simulink model "test_emplanner_cs_old"  (R2021a)
settings: Solver=ode5  StartTime=0.0  StopTime=120  FixedStep=1/1000  RelTol=1e-3
PreLoadFcn:
  | mbxruntime.callbacks.PreLoadFcn(bdroot);
PostLoadFcn:
  | mbxruntime.callbacks.PostLoadFcn(bdroot);
InitFcn:
  | mbxruntime.callbacks.InitFcn(bdroot);
StartFcn:
  | mbxruntime.callbacks.StartFcn(bdroot);
StopFcn:
  | mbxruntime.callbacks.StopFcn(bdroot);
model workspace (MAT data in the model file):
  mbox_table : object (value not decoded)
  model_closed = 0
  sim_status = 0
values from neighbouring files (symbols this model uses):
  c_factor = 43.75    [emplanner_init.m]
  cf = -175016    [emplanner_init.m]
  cr = -130634    [emplanner_init.m]
  global_path_x = [-2.7494 -1.75001774493 -0.751894634419 0.244952249347 1.24051712279 2.23479835808 3.22779585569 4.21951007764 5.20994169183 6.19909144113 7.18696009523 8.17354843293 ... (3001 elements, 3001x1)]    [global_path.mat]
  global_path_y = [18.2589 18.2589 18.2589 18.2589 18.2589 18.2589 18.2589 18.2589 18.2589 18.2589 18.2589 18.2589 ... (3001 elements, 3001x1)]    [global_path.mat]
  KD_PID_distance = 0.0    (= 0)    [emplanner_init.m]
  KD_PID_speed = 0    [emplanner_init.m]
  KI_PID_distance = 0.0    (= 0)    [emplanner_init.m]
  KI_PID_speed = 0    [emplanner_init.m]
  KP_PID_distance = 0.5    [emplanner_init.m]
  KP_PID_speed = 1.8    [emplanner_init.m]
  la = 1.265    [emplanner_init.m]
  lb = 2.947-1.265    (= 1.682)    [emplanner_init.m]
  LQR_K1 = k(:,1)'    [emplanner_init.m]
  LQR_K2 = k(:,2)'    [emplanner_init.m]
  LQR_K3 = k(:,3)'    [emplanner_init.m]
  LQR_K4 = k(:,4)'    [emplanner_init.m]
  m = 2020    [emplanner_init.m]
  rack_displacement = [-39.14 , -37.2 , -35.29 , -33.43 , -31.6 , -29.81 , -28.06 , -26.34 , -24.66 ,      -23.01 , -21.38 , -19.79 , -18.23 , -16.69 , -15.18 , -13.7 , -12.23 , -10.8 , -9.38 , -7.98 ,     -6.61 , -5.25 , -3.91 , -2.59 , -1.29 , 0 , 1.27 , 2.54 , 3.78 , 5.02 , 6.24 , 7.46 , 8.66 ,      9.86 , 11.05 , 12.24 , 13.41 , 14.59 , 15.76 , 16.92 , 18.09 , 19.25 , 20.42 , 21.59 , 22.76 ,      23.93 , 25.11 , 26 ...(+26 chars)    [emplanner_init.m]
  right_wheel_ground = [-70 ,-67.2 , -64.4 , -61.6 , -58.8 , -56 , -53.2 , -50.4 , -47.6 , -44.8 , -42 ,      -39.2 , -36.4 , -33.6 , -30.8 , -28 , -25.2 , -22.4 , -19.6 , -16.8 , -14 , -11.2 , -8.4 , -5.6 ,      -2.8 , 0 , 2.8 , 5.6 , 8.4 , 11.2 , 14 , 16.8 , 19.6 , 22.4 , 25.2 , 28 , 30.8 , 33.6 , 36.4 ,      39.2 , 42 , 44.8 , 47.6 , 50.4 , 53.2 , 56 , 58.8 , 61.6 , 64.4 , 67.2 , 70 ]    [emplanner_init.m]
  vx_break_point = zeros(1,5000)    [emplanner_init.m]
undefined symbols (not defined in the file or in its folder): aubr, DiscIntNeverNeededParam, tablebr, vubr, warningInitialVelocity, x0
libraries: PreScanSimulinkLibrary x27, simulink x19, simulink_extras x6, Solver_SF x1
(part 5 of 11)

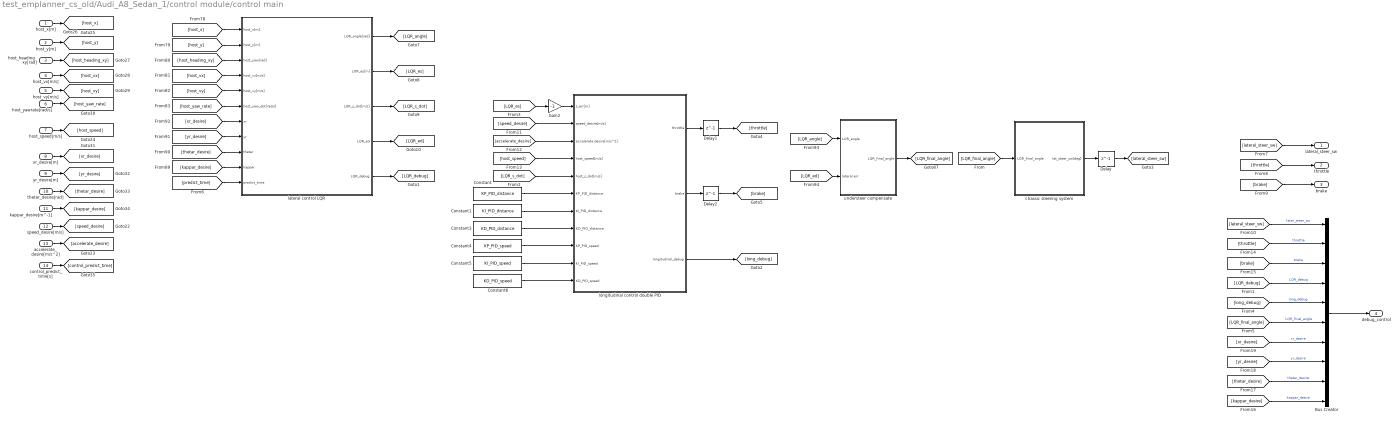
== system test_emplanner_cs_old/Audi_A8_Sedan_1/control module/control main ==
  host_x[m] : Inport
  host_y[m] : Inport  Port=2
  host_heading_xy[rad] : Inport  Port=3
  host_vx[m/s] : Inport  Port=4
  host_vy[m/s] : Inport  Port=5
  host_yawrate[rad/s] : Inport  Port=6
  host_speed[m/s] : Inport  Port=7
  xr_desire[m] : Inport  Port=8
  yr_desire[m] : Inport  Port=9
  thetar_desire[rad] : Inport  Port=10
  kappar_desire[m^-1] : Inport  Port=11
  speed_desire[m/s] : Inport  Port=12
  accelerate_desire[m/s^2] : Inport  Port=13
  control_predict_time[s] : Inport  Port=14
  Bus Creator : BusCreator  Inputs=10
  Constant : Constant  Value=KP_PID_distance
  Constant1 : Constant  Value=KI_PID_distance
  Constant3 : Constant  Value=KD_PID_distance
  Constant4 : Constant  Value=KP_PID_speed
  Constant5 : Constant  Value=KI_PID_speed
  Constant6 : Constant  Value=KD_PID_speed
  Delay : Delay  DelayLength=1
  Delay1 : Delay  DelayLength=1
  Delay2 : Delay  DelayLength=1
  Gain2 : Gain  Gain=-1
  chassic steering system : Subsystem
  lateral control LQR : Subsystem
  longitudinal control double PID : Subsystem
  understeer compensate : Subsystem
  lateral_steer_sw : Outport
  throttle : Outport  Port=2
  brake : Outport  Port=3
  debug_control : Outport  Port=4
  wires:
  host_x[m]/1 -> [host_x]
  understeer compensate/1(LQR_final_angle) -> [LQR_final_angle]
  lateral control LQR/1(LQR_angle[rad]) -> [LQR_angle]
  [host_vx] -> lateral control LQR/4(host_vx[m/s])
  thetar_desire[rad]/1 -> [thetar_desire]
  Constant1/1 -> longitudinal control double PID/7(KI_PID_distance)
  [accelerate_desire] -> longitudinal control double PID/3(accelerate desire[m/s^2])
  [host_x] -> lateral control LQR/1(host_x[m])
  [xr_desire] -> lateral control LQR/7(xr)
  accelerate_desire[m/s^2]/1 -> [accelerate_desire]
  [host_y] -> lateral control LQR/2(host_y[m])
  [LQR_s_dot] -> longitudinal control double PID/5(host_s_dot[m/s])
  [yr_desire] -> lateral control LQR/8(yr)
  [LQR_angle] -> understeer compensate/1(LQR_angle)
  xr_desire[m]/1 -> [xr_desire]
  [host_vy] -> lateral control LQR/5(host_vy[m/s])
  lateral control LQR/2(LQR_es[m]) -> [LQR_es]
  host_heading_xy[rad]/1 -> [host_heading_xy]
  [LQR_ed] -> understeer compensate/2(lateral err)
  lateral control LQR/3(LQR_s_dot[m/s]) -> [LQR_s_dot]
  Constant/1 -> longitudinal control double PID/6(KP_PID_distance)
  Constant3/1 -> longitudinal control double PID/8(KD_PID_distance)
  Constant5/1 -> longitudinal control double PID/10(KI_PID_speed)
  Constant4/1 -> longitudinal control double PID/9(KP_PID_speed)
  [host_speed] -> longitudinal control double PID/4(host_speed[m/s])
  [predict_time] -> lateral control LQR/11(predict_time)
  host_vx[m/s]/1 -> [host_vx]
  [speed_desire] -> longitudinal control double PID/2(speed_desire[m/s])
  lateral control LQR/4(LQR_ed) -> [LQR_ed]
  [thetar_desire] -> lateral control LQR/9(thetar)
  [host_heading_xy] -> lateral control LQR/3(host_yaw[rad])
  [kappar_desire] -> lateral control LQR/10(kappar)
  host_yawrate[rad/s]/1 -> [host_yaw_rate]
  kappar_desire[m^-1]/1 -> [kappar_desire]
  yr_desire[m]/1 -> [yr_desire]
  [host_yaw_rate] -> lateral control LQR/6(host_yaw_dot[rad/s])
  host_y[m]/1 -> [host_y]
  host_vy[m/s]/1 -> [host_vy]
  host_speed[m/s]/1 -> [host_speed]
  control_predict_time[s]/1 -> [control_predict_time]
  speed_desire[m/s]/1 -> [speed_desire]
  Constant6/1 -> longitudinal control double PID/11(KD_PID_speed)
  Gain2/1 -> longitudinal control double PID/1(s_err[m])
  [LQR_es] -> Gain2/1
  [LQR_final_angle] -> chassic steering system/1(LQR_final_angle)
  chassic steering system/1(lat_steer_sw[deg]) -> Delay/1
  longitudinal control double PID/1(throttle) -> Delay1/1
  longitudinal control double PID/2(brake) -> Delay2/1
  lateral control LQR/5(LQR_debug) -> [LQR_debug]
  longitudinal control double PID/3(longitudinal_debug) -> [long_debug]
  Delay/1 -> [lateral_steer_sw]
  Delay1/1 -> [throttle]
  Delay2/1 -> [brake]
  [lateral_steer_sw] -> lateral_steer_sw/1
  [throttle] -> throttle/1
  [brake] -> brake/1
  [lateral_steer_sw] -> Bus Creator/1  "later_steer_sw"
  [throttle] -> Bus Creator/2  "throttle"
  [brake] -> Bus Creator/3  "brake"
  [LQR_debug] -> Bus Creator/4  "LQR_debug"
  [long_debug] -> Bus Creator/5  "long_debug"
  [LQR_final_angle] -> Bus Creator/6  "LQR_final_angle"
  Bus Creator/1 -> debug_control/1
  [xr_desire] -> Bus Creator/7  "xr_desire"
  [yr_desire] -> Bus Creator/8  "yr_desire"
  [thetar_desire] -> Bus Creator/9  "thetar_desire"
  [kappar_desire] -> Bus Creator/10  "kappar_desire"

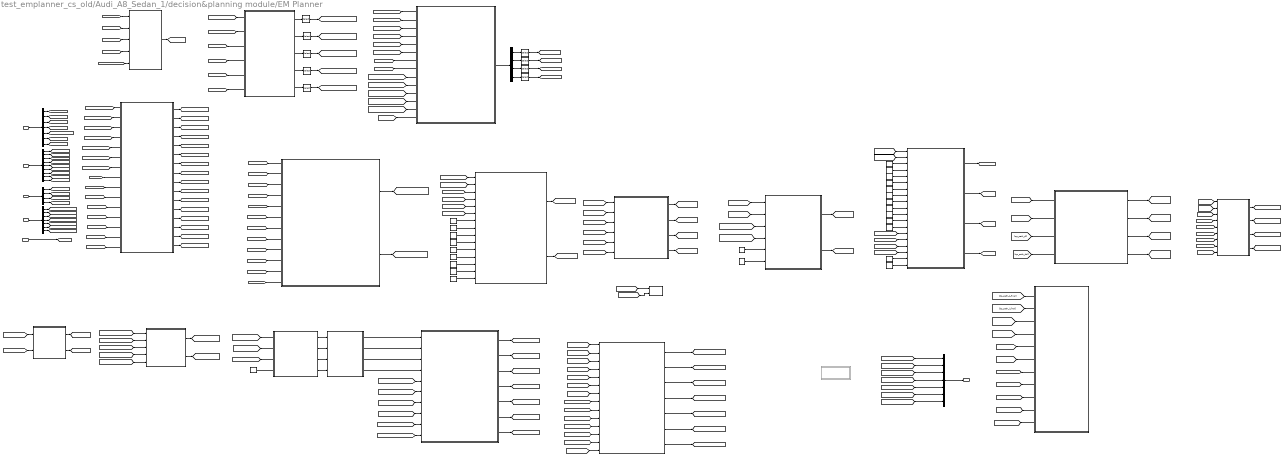
== system test_emplanner_cs_old/Audi_A8_Sedan_1/decision&planning module/EM Planner ==
  reference info : Inport
  location info : Inport  Port=2
  perception info : Inport  Port=3
  pre_planning info : Inport  Port=4
  current time : Inport  Port=5
  " frenet2cartesian" : MATLAB Function  TreatAsAtomicUnit=on
  Bus Creator : BusCreator  Inputs=7
  Bus Selector : BusSelector  OutputSignals=referenceline_x,referenceline_y,reference_heading,reference_kappa,origin_match_point_index,origin_x,origin_y
  Bus Selector1 : BusSelector  OutputSignals=host_x,host_y,host_heading_xy,host_vx,host_vy,host_yawrate,host_speed,host_ax,host_ay
  Bus Selector2 : BusSelector  OutputSignals=obs_x_set_gcs,obs_y_set_gcs,obs_velocity_set_gcs,obs_heading_set_gcs
  Bus Selector3 : BusSelector  OutputSignals=trajectory_x_gcs,trajectory_y_gcs,trajectory_heading_gcs,trajectory_kappa_gcs,trajectory_speed_gcs,trajectory_accel_gcs,trajectory_time_gcs
  Bus Selector4 : BusSelector  OutputSignals=s_set,l_set,dl_set,ddl_set
  Constant : Constant  Value=1e8
  Constant1 : Constant  Value=300
  Constant10 : Constant  Value=5
  Constant11 : Constant  Value=2
  Constant12 : Constant  Value=1.63
  Constant13 : Constant  Value=3
  Constant14 : Constant  Value=3
  Constant15 : Constant  Value=5
  Constant16 : Constant  Value=50000
  Constant17 : Constant  Value=300
  Constant18 : Constant  Value=15
  Constant19 : Constant  Value=1200
  Constant2 : Constant  Value=2000
  Constant20 : Constant  Value=40
  Constant21 : Constant  Value=40
  Constant22 : Constant  Value=40
  Constant23 : Constant  Value=0.1
  Constant24 : Constant  Value=0.02
  Constant3 : Constant  Value=10000
  Constant4 : Constant  Value=20
  Constant5 : Constant  Value=9
  Constant6 : Constant  Value=4
  Constant7 : Constant  Value=15
  Constant8 : Constant
  Constant9 : Constant  Value=8
  MATLAB Function : MATLAB Function  TreatAsAtomicUnit=on
  MATLAB Function1 : MATLAB Function  TreatAsAtomicUnit=on
  MATLAB Function2 : MATLAB Function  Commented=on  TreatAsAtomicUnit=on
  Selector{1..9} (9 alike) : Selector  InputPortWidth=128  IndexOptions=Index vector (dialog)  Indices=1  OutputSizes=1
  calc path length and map between point and s : MATLAB Function  TreatAsAtomicUnit=on
  calc plan start info and stitch_trajectory : MATLAB Function  TreatAsAtomicUnit=on
  calc speed planning start condition : MATLAB Function  TreatAsAtomicUnit=on
  cartesian2frenet : Subsystem
  generate convex space : MATLAB Function  TreatAsAtomicUnit=on
  increase DP path nodes : MATLAB Function  TreatAsAtomicUnit=on
  increase st point count : MATLAB Function  TreatAsAtomicUnit=on
  index2s : MATLAB Function  TreatAsAtomicUnit=on
  mine_tou : MATLAB Function  TreatAsAtomicUnit=on
  obs : Subsystem
  path and speed merge : MATLAB Function  TreatAsAtomicUnit=on
  path desion with dynamic planning(dp) : MATLAB Function  TreatAsAtomicUnit=on
  plot : MATLAB Function  TreatAsAtomicUnit=on
  qp : MATLAB Function  TreatAsAtomicUnit=on
  simple speed qp planning : MATLAB Function  TreatAsAtomicUnit=on
  stitch trajectory : MATLAB Function  TreatAsAtomicUnit=on
  EM Planner result : Outport
  wires:
  reference info/1 -> Bus Selector/1
  location info/1 -> Bus Selector1/1
  perception info/1 -> Bus Selector2/1
  pre_planning info/1 -> Bus Selector3/1
  current time/1 -> [current_time]
  Bus Selector3/1 -> [pre_trajectory_x_gcs]  "<trajectory_x_gcs>"
  Bus Selector2/1 -> [obs_x_set_gcs]  "<obs_x_set_gcs>"
  Bus Selector2/2 -> [obs_y_set_gcs]  "<obs_y_set_gcs>"
  Bus Selector2/3 -> [obs_velocity_set_gcs]  "<obs_velocity_set_gcs>"
  Bus Selector2/4 -> [obs_heading_set_gcs]  "<obs_heading_set_gcs>"
  Bus Selector1/1 -> [host_x]  "<host_x>"
  Bus Selector1/2 -> [host_y]  "<host_y>"
  Bus Selector1/3 -> [host_heading_xy]  "<host_heading_xy>"
  Bus Selector1/4 -> [host_vx_vcs]  "<host_vx>"
  Bus Selector1/5 -> [host_vy_vcs]  "<host_vy>"
  Bus Selector1/6 -> [host_yawrate]  "<host_yawrate>"
  Bus Selector1/7 -> [host_speed]  "<host_speed>"
  Bus Selector1/8 -> [host_ax_vcs]  "<host_ax>"
  Bus Selector1/9 -> [host_ay_vcs]  "<host_ay>"
  Bus Selector/1 -> [referenceline_x]  "<referenceline_x>"
  Bus Selector/2 -> [referenceline_y]  "<referenceline_y>"
  Bus Selector/3 -> [referenceline_heading]  "<reference_heading>"
  Bus Selector/4 -> [referenceline_kappa]  "<reference_kappa>"
  [pre_trajectory_x_gcs] -> calc plan start info and stitch_trajectory/1(pre_trajectory_x)
  [pre_trajectory_y_gcs] -> calc plan start info and stitch_trajectory/2(pre_trajectory_y)
  [pre_trajectory_heading_gcs] -> calc plan start info and stitch_trajectory/3(pre_trajectory_heading)
  [pre_trajectory_kappa_gcs] -> calc plan start info and stitch_trajectory/4(pre_trajectory_kappa)
  [pre_trajectory_speed_gcs] -> calc plan start info and stitch_trajectory/5(pre_trajectory_velocity)
  [pre_trajectory_accel_gcs] -> calc plan start info and stitch_trajectory/6(pre_trajectory_accel)
  [pre_trajectory_time] -> calc plan start info and stitch_trajectory/7(pre_trajectory_time)
  [current_time] -> calc plan start info and stitch_trajectory/8(current_time)
  [host_x] -> calc plan start info and stitch_trajectory/9(host_x)
  [host_y] -> calc plan start info and stitch_trajectory/10(host_y)
  [host_heading_xy] -> calc plan start info and stitch_trajectory/11(host_heading_xy)
  [host_vx_vcs] -> calc plan start info and stitch_trajectory/12(host_vx)
  [host_vy_vcs] -> calc plan start info and stitch_trajectory/13(host_vy)
  [host_ax_vcs] -> calc plan start info and stitch_trajectory/14(host_ax)
  [host_ay_vcs] -> calc plan start info and stitch_trajectory/15(host_ay)
  calc plan start info and stitch_trajectory/1(plan_start_x) -> [plan_start_x_gcs]
  calc plan start info and stitch_trajectory/2(plan_start_y) -> [plan_start_y_gcs]
  calc plan start info and stitch_trajectory/3(plan_start_heading) -> [plan_start_heading_gcs]
  calc plan start info and stitch_trajectory/4(plan_start_kappa) -> [plan_start_kappa_gcs]
  calc plan start info and stitch_trajectory/5(plan_start_vx) -> [plan_start_vx_gcs]
  calc plan start info and stitch_trajectory/6(plan_start_vy) -> [plan_start_vy_gcs]
  calc plan start info and stitch_trajectory/7(plan_start_ax) -> [plan_start_ax_gcs]
  calc plan start info and stitch_trajectory/8(plan_start_ay) -> [plan_start_ay_gcs]
  calc plan start info and stitch_trajectory/9(plan_start_time) -> [plan_start_time]
  calc plan start info and stitch_trajectory/10(stitch_x) -> [stitch_x_gcs]
  calc plan start info and stitch_trajectory/11(stitch_y) -> [stitch_y_gcs]
  calc plan start info and stitch_trajectory/12(stitch_heading) -> [stitch_heading_gcs]
  calc plan start info and stitch_trajectory/13(stitch_kappa) -> [stitch_kappa_gcs]
  calc plan start info and stitch_trajectory/14(stitch_speed) -> [stitch_speed_gcs]
  calc plan start info and stitch_trajectory/15(stitch_accel) -> [stitch_accel_gcs]
  calc plan start info and stitch_trajectory/16(stitch_time) -> [stitch_time]
  Bus Selector/5 -> [origin_match_point_index]  "<origin_match_point_index>"
  Bus Selector/6 -> [origin_x]  "<origin_x>"
  Bus Selector/7 -> [origin_y]  "<origin_y>"
  [referenceline_x] -> index2s/1(path_x)
  [referenceline_y] -> index2s/2(path_y)
  [origin_x] -> index2s/3(origin_x)
  [origin_y] -> index2s/4(origin_y)
  [origin_match_point_index] -> index2s/5(origin_match_point_index)
  index2s/1(index2s) -> [index2s]
  mine_tou/5(proj_kappa_set) -> Selector5/1
  mine_tou/1(match_point_index_set) -> Selector1/1
  mine_tou/4(proj_heading_set) -> Selector4/1
  mine_tou/2(proj_x_set) -> Selector2/1
  mine_tou/3(proj_y_set) -> Selector3/1
  [plan_start_x_gcs] -> mine_tou/1(x_set)
  [plan_start_y_gcs] -> mine_tou/2(y_set)
  [referenceline_x] -> mine_tou/3(frenet_path_x_set)
  [referenceline_y] -> mine_tou/4(frenet_path_y_set)
  [referenceline_kappa] -> mine_tou/6(frenet_path_kappa_set)
  [referenceline_heading] -> mine_tou/5(frenet_path_heading_set)
  Selector1/1 -> [plan_start_match_point_index]
  Selector2/1 -> [plan_start_proj_x]
  Selector3/1 -> [plan_start_proj_y]
  Selector4/1 -> [plan_start_proj_heading]
  Selector5/1 -> [plan_start_proj_kappa]
  [plan_start_x_gcs] -> cartesian2frenet/1(x_set)
  [plan_start_y_gcs] -> cartesian2frenet/2(y_set)
  [plan_start_vx_gcs] -> cartesian2frenet/3(vx_set)
  [plan_start_vy_gcs] -> cartesian2frenet/4(vy_set)
  [plan_start_ax_gcs] -> cartesian2frenet/5(ax_set)
  [plan_start_ay_gcs] -> cartesian2frenet/6(ay_set)
  [referenceline_x] -> cartesian2frenet/7(frenet_path_x)
  [referenceline_y] -> cartesian2frenet/8(frenet_path_y)
  [plan_start_match_point_index] -> cartesian2frenet/9(proj_match_point_index_set)
  [plan_start_proj_x] -> cartesian2frenet/10(proj_x_set)
  [plan_start_proj_y] -> cartesian2frenet/11(proj_y_set)
  [plan_start_proj_heading] -> cartesian2frenet/12(proj_heading_set)
  [plan_start_proj_kappa] -> cartesian2frenet/13(proj_kappa_set)
  [index2s] -> cartesian2frenet/14(index2s)
  cartesian2frenet/1(cartesian2frenetout) -> Bus Selector4/1
  Bus Selector4/1 -> Selector6/1  "<s_set>"
  Selector6/1 -> [plan_start_s]
  Bus Selector4/2 -> Selector7/1  "<l_set>"
  Selector7/1 -> [plan_start_l]
  Bus Selector4/3 -> Selector8/1  "<dl_set>"
  Selector8/1 -> [plan_start_dl]
  Bus Selector4/4 -> Selector9/1  "<ddl_set>"
  Selector9/1 -> [plan_start_ddl]
  [host_x] -> obs/1(host_x)
  [host_y] -> obs/2(host_y)
  [host_heading_xy] -> obs/3(host_heading_xy)
  [obs_x_set_gcs] -> obs/4(obs_x_set_gcs)
  [obs_y_set_gcs] -> obs/5(obs_y_set_gcs)
  [obs_velocity_set_gcs] -> obs/6(obs_velocity_set_gcs)
  [obs_heading_set_gcs] -> obs/7(obs_heading_set_gcs)
  [referenceline_x] -> obs/8(referenceline_x)
  [referenceline_y] -> obs/9(referenceline_y)
  [referenceline_heading] -> obs/10(referenceline_heading)
  [referenceline_kappa] -> obs/11(referenceline_kappa)
  [index2s] -> obs/12(index2s)
  obs/1(static_obs_s_set) -> [static_obs_s_set]
  obs/2(static_obs_l_set) -> [static_obs_l_set]
  [static_obs_s_set] -> path desion with dynamic planning(dp)/1(obs_s_set)
  [static_obs_l_set] -> path desion with dynamic planning(dp)/2(obs_l_set)
  [plan_start_s] -> path desion with dynamic planning(dp)/3(plan_start_s)
  [plan_start_l] -> path desion with dynamic planning(dp)/4(plan_start_l)
  [plan_start_dl] -> path desion with dynamic planning(dp)/5(plan_start_dl)
  [plan_start_ddl] -> path desion with dynamic planning(dp)/6(plan_start_dll)
  Constant/1 -> path desion with dynamic planning(dp)/7(w_cost_collision)
  Constant1/1 -> path desion with dynamic planning(dp)/8(w_cost_smooth_dl)
  Constant2/1 -> path desion with dynamic planning(dp)/9(w_cost_smooth_ddl)
  Constant3/1 -> path desion with dynamic planning(dp)/10(w_cost_smooth_dddl)
  Constant4/1 -> path desion with dynamic planning(dp)/11(w_cost_ref)
  Constant5/1 -> path desion with dynamic planning(dp)/12(row)
  Constant6/1 -> path desion with dynamic planning(dp)/13(col)
  Constant7/1 -> path desion with dynamic planning(dp)/14(sample_s)
  Constant8/1 -> path desion with dynamic planning(dp)/15(sample_l)
  path desion with dynamic planning(dp)/1(dp_path_s) -> [dp_path_s_init]
  path desion with dynamic planning(dp)/2(dp_path_l) -> [dp_path_l_init]
  [dp_path_s_init] -> increase DP path nodes/1(dp_path_s_init)
  [dp_path_l_init] -> increase DP path nodes/2(dp_path_l_init)
  [plan_start_s] -> increase DP path nodes/3(plan_start_s)
  [plan_start_dl] -> increase DP path nodes/5(plan_start_dl)
  [plan_start_ddl] -> increase DP path nodes/6(plan_start_ddl)
  increase DP path nodes/1(dp_path_s_final) -> [dp_path_s_final]
  increase DP path nodes/2(dp_path_l_final) -> [dp_path_l_final]
  increase DP path nodes/3(dp_path_dl_final) -> [dp_path_dl_final]
  increase DP path nodes/4(dp_path_ddl_final) -> [dp_path_ddl_final]
  [qp_path_s_final] -> " frenet2cartesian"/1(s_set)
  [qp_path_l_final] -> " frenet2cartesian"/2(l_set)
  [qp_path_dl_final] -> " frenet2cartesian"/3(dl_set)
  [qp_path_ddl_final] -> " frenet2cartesian"/4(ddl_set)
  [plan_start_l] -> increase DP path nodes/4(plan_start_l)
  " frenet2cartesian"/1(x_set) -> [trajectory_x_init]
  " frenet2cartesian"/4(kappa_set) -> [trajectory_kappa_init]
  " frenet2cartesian"/3(heading_set) -> [trajectory_heading_init]
  " frenet2cartesian"/2(y_set) -> [trajectory_y_init]
  [trajectory_heading_init] -> path and speed merge/9(trajectory_heading_init)
  stitch trajectory/7(trajectory_time_final) -> [trajectory_time_final]
  [plan_start_time] -> path and speed merge/5(current_time)
  [trajectory_heading] -> stitch trajectory/3(trajectory_heading)
  [trajectory_x_init] -> calc path length and map between point and s/1(trajectory_x)
  increase st point count/3(s_dot2) -> path and speed merge/3(s_dot2)
  [path_s_end] -> simple speed qp planning/3(s_end)
  [trajectory_x_init] -> path and speed merge/7(trajectory_x_init)
  increase st point count/4(relative_time) -> path and speed merge/4(relative_time)
  [stitch_kappa_gcs] -> stitch trajectory/11(stitch_kappa)
  [trajectory_x] -> stitch trajectory/1(trajectory_x)
  [trajectory_y_init] -> path and speed merge/8(trajectory_y_init)
  stitch trajectory/4(trajectory_kappa_final) -> [trajectory_kappa_final]
  simple speed qp planning/2(s_dot_init) -> increase st point count/2(s_dot_init)
  [trajectory_y] -> stitch trajectory/2(trajectory_y)
  [trajectory_time] -> stitch trajectory/7(trajectory_time)
  Constant9/1 -> simple speed qp planning/4(recommend_T)
  simple speed qp planning/1(s_init) -> increase st point count/1(s_init)
  [plan_start_ay_gcs] -> calc speed planning start condition/4(plan_start_ay)
  calc path length and map between point and s/1(path_s_end) -> [path_s_end]
  path and speed merge/6(trajectory_accel) -> [trajectory_accel]
  increase st point count/1(s) -> path and speed merge/1(s)
  simple speed qp planning/4(relative_time_init) -> increase st point count/4(relative_time_init)
  [trajectory_y_init] -> calc path length and map between point and s/2(trajectory_y)
  [stitch_y_gcs] -> stitch trajectory/9(stitch_y)
  [trajectory_kappa_init] -> path and speed merge/10(trajectory_kappa_init)
  increase st point count/2(s_dot) -> path and speed merge/2(s_dot)
  calc path length and map between point and s/2(path_s) -> [path_s]
  calc speed planning start condition/1(plan_start_s_dot) -> [plan_start_s_dot]
  path and speed merge/2(trajectory_y) -> [trajectory_y]
  [trajectory_kappa] -> stitch trajectory/4(trajectory_kappa)
  simple speed qp planning/3(s_dot2_init) -> increase st point count/3(s_dot2_init)
  path and speed merge/3(trajectory_heading) -> [trajectory_heading]
  path and speed merge/1(trajectory_x) -> [trajectory_x]
  path and speed merge/5(trajectory_speed) -> [trajectory_speed]
  stitch trajectory/5(trajectory_speed_final) -> [trajectory_speed_final]
  [stitch_time] -> stitch trajectory/14(stitch_time)
  stitch trajectory/6(trajectory_accel_final) -> [trajectory_accel_final]
  [stitch_accel_gcs] -> stitch trajectory/13(stitch_accel)
  [trajectory_speed] -> stitch trajectory/5(trajectory_speed)
  path and speed merge/4(trajectory_kappa) -> [trajectory_kappa]
  [plan_start_vy_gcs] -> calc speed planning start condition/2(plan_start_vy)
  [plan_start_heading_gcs] -> calc speed planning start condition/5(plan_start_heading)
  calc speed planning start condition/2(plan_start_s_dot2) -> [plan_start_s_dot2]
  [plan_start_s_dot2] -> simple speed qp planning/2(plan_start_s_dot2)
  stitch trajectory/1(trajectory_x_final) -> [trajectory_x_final]
  [stitch_speed_gcs] -> stitch trajectory/12(stitch_speed)
  [stitch_heading_gcs] -> stitch trajectory/10(stitch_heading)
  [plan_start_s_dot] -> simple speed qp planning/1(plan_start_s_dot)
  [trajectory_accel] -> stitch trajectory/6(trajectory_accel)
  [plan_start_vx_gcs] -> calc speed planning start condition/1(plan_start_vx)
  stitch trajectory/2(trajectory_y_final) -> [trajectory_y_final]
  [plan_start_ax_gcs] -> calc speed planning start condition/3(plan_start_ax)
  stitch trajectory/3(trajectory_heading_final) -> [trajectory_heading_final]
  path and speed merge/7(trajectory_time) -> [trajectory_time]
  [stitch_x_gcs] -> stitch trajectory/8(stitch_x)
  [path_s] -> path and speed merge/6(path_s)
  [trajectory_speed_final] -> Bus Creator/5  "trajectory_speed_gcs"
  [trajectory_y_final] -> Bus Creator/2  "trajectory_y_gcs"
  Bus Creator/1 -> EM Planner result/1
  [trajectory_kappa_final] -> Bus Creator/4  "trajectory_kappa_gcs"
  [trajectory_accel_final] -> Bus Creator/6  "trajectory_accel_gcs"
  [trajectory_time_final] -> Bus Creator/7  "trajectory_time_gcs"
  [trajectory_x_final] -> Bus Creator/1  "trajectory_x_gcs"
  Bus Selector3/2 -> [pre_trajectory_y_gcs]  "<trajectory_y_gcs>"
  Bus Selector3/3 -> [pre_trajectory_heading_gcs]  "<trajectory_heading_gcs>"
  Bus Selector3/4 -> [pre_trajectory_kappa_gcs]  "<trajectory_kappa_gcs>"
  Bus Selector3/5 -> [pre_trajectory_speed_gcs]  "<trajectory_speed_gcs>"
  Bus Selector3/6 -> [pre_trajectory_accel_gcs]  "<trajectory_accel_gcs>"
  Bus Selector3/7 -> [pre_trajectory_time]  "<trajectory_time_gcs>"
  [dp_path_s_final] -> MATLAB Function/1(s)
  [dp_path_l_final] -> MATLAB Function/2(l)
  [dp_path_s_final] -> generate convex space/1(dp_path_s)
  [dp_path_l_final] -> generate convex space/2(dp_path_l)
  [static_obs_s_set] -> generate convex space/3(static_obs_s_set)
  [static_obs_l_set] -> generate convex space/4(static_obs_l_set)
  Constant10/1 -> generate convex space/5(static_obs_length)
  Constant11/1 -> generate convex space/6(static_obs_width)
  generate convex space/1(l_min) -> [l_min]
  generate convex space/2(l_max) -> [l_max]
  [plan_start_l] -> qp/15(plan_start_l)
  [plan_start_dl] -> qp/16(plan_start_dl)
  [plan_start_ddl] -> qp/17(plan_start_ddl)
  Constant12/1 -> qp/13(host_w)
  Constant13/1 -> qp/12(host_d2)
  Constant14/1 -> qp/11(host_d1)
  [l_min] -> qp/1(l_min)
  [l_max] -> qp/2(l_max)
  Constant15/1 -> qp/3(w_cost_l)
  Constant16/1 -> qp/4(w_cost_dl)
  Constant17/1 -> qp/5(w_cost_ddl)
  Constant18/1 -> qp/6(w_cost_dddl)
  Constant19/1 -> qp/7(w_cost_centre)
  Constant20/1 -> qp/8(w_cost_end_l)
  Constant21/1 -> qp/9(w_cost_end_dl)
  Constant22/1 -> qp/10(w_cost_end_ddl)
  qp/2(qp_path_l) -> [qp_path_l]
  qp/3(qp_path_dl) -> [qp_path_dl]
  qp/4(qp_path_ddl) -> [qp_path_ddl]
  [referenceline_x] -> " frenet2cartesian"/5(frenet_path_x)
  [referenceline_y] -> " frenet2cartesian"/6(frenet_path_y)
  [referenceline_heading] -> " frenet2cartesian"/7(frenet_path_heading)
  [referenceline_kappa] -> " frenet2cartesian"/8(frenet_path_kappa)
  [index2s] -> " frenet2cartesian"/9(index2s)
  [plan_start_l] -> plot/10(start_l)
  [static_obs_l_set] -> plot/8(obs_l_set)
  [l_max] -> plot/6(l_max)
  [static_obs_s_set] -> plot/7(obs_s_set)
  [plan_start_dl] -> plot/11(start_dl)
  [plan_start_s] -> plot/9(start_s)
  [l_min] -> plot/5(l_min)
  [dp_path_l_final] -> plot/2(dp_l)
  [dp_path_s_final] -> plot/1(dp_s)
  [plan_start_s] -> qp/14(plan_start_s)
  Constant24/1 -> qp/19(delta_ddl_max)
  Constant23/1 -> qp/18(delta_dl_max)
  MATLAB Function1/1(qp_path_s_final) -> [qp_path_s_final]
  [qp_path_s] -> MATLAB Function1/1(qp_path_s)
  MATLAB Function1/4(qp_path_ddl_final) -> [qp_path_ddl_final]
  MATLAB Function1/3(qp_path_dl_final) -> [qp_path_dl_final]
  [qp_path_ddl] -> MATLAB Function1/4(qp_path_ddl)
  [qp_path_dl] -> MATLAB Function1/3(qp_path_dl)
  [qp_path_l] -> MATLAB Function1/2(qp_path_l)
  MATLAB Function1/2(qp_path_l_final) -> [qp_path_l_final]
  qp/1(qp_path_s) -> [qp_path_s]
  [qp_path_s_final] -> plot/3(qp_s)
  [qp_path_l_final] -> plot/4(qp_l)
  [trajectory_heading_final] -> Bus Creator/3  "trajectory_heading_gcs"

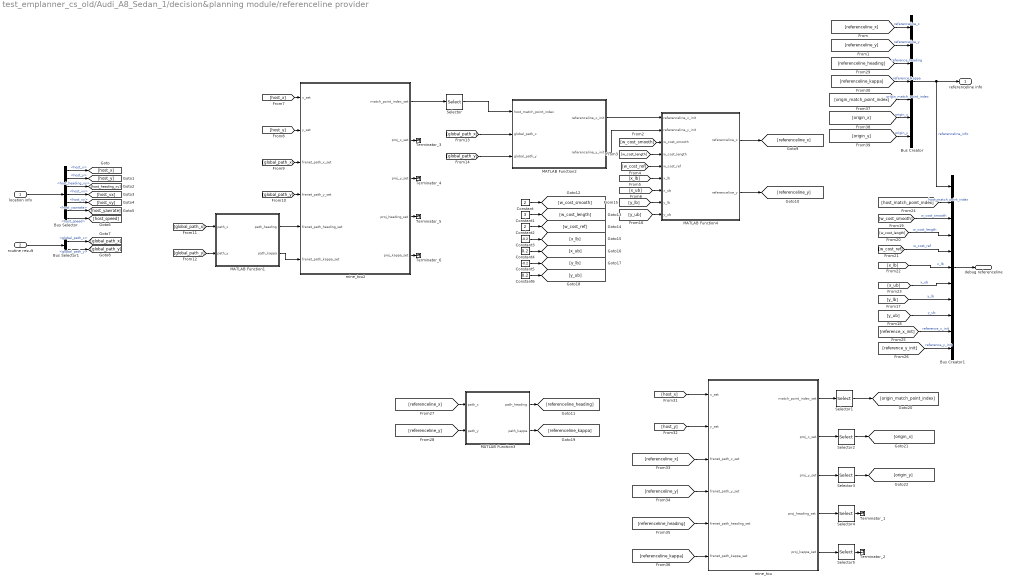
== system test_emplanner_cs_old/Audi_A8_Sedan_1/decision&planning module/referenceline provider ==
  location info : Inport
  routine result : Inport  Port=2
  Bus Creator : BusCreator  Inputs=7
  Bus Creator1 : BusCreator  Inputs=11
  Bus Selector : BusSelector  OutputSignals=host_x,host_y,host_heading_xy,host_vx,host_vy,host_yawrate,host_speed
  Bus Selector1 : BusSelector  OutputSignals=global_path_x,global_path_y
  Constant : Constant  Value=2
  Constant1 : Constant  Value=3
  Constant2 : Constant  Value=2
  Constant3 : Constant  Value=-0.2
  Constant4 : Constant  Value=0.2
  Constant5 : Constant  Value=-0.2
  Constant6 : Constant  Value=0.2
  MATLAB Function1 : MATLAB Function  TreatAsAtomicUnit=on
  MATLAB Function2 : MATLAB Function  TreatAsAtomicUnit=on
  MATLAB Function3 : MATLAB Function  TreatAsAtomicUnit=on
  MATLAB Function4 : MATLAB Function  TreatAsAtomicUnit=on
  Selector{,1..5} (6 alike) : Selector  InputPortWidth=128  IndexOptions=Index vector (dialog)  Indices=1  OutputSizes=1
  Terminator_{1..6} (6 alike) : Terminator
  mine_tou : MATLAB Function  TreatAsAtomicUnit=on
  mine_tou2 : MATLAB Function  TreatAsAtomicUnit=on
  referenceline info : Outport
  debug referenceline : Outport  Port=2
  wires:
  [global_path_x] -> MATLAB Function1/1(path_x)
  Selector/1 -> MATLAB Function2/1(host_match_point_index)
  MATLAB Function1/1(path_heading) -> mine_tou2/5(frenet_path_heading_set)
  MATLAB Function1/2(path_kappa) -> mine_tou2/6(frenet_path_kappa_set)
  [global_path_y] -> MATLAB Function2/3(global_path_y)
  [global_path_y] -> MATLAB Function1/2(path_y)
  MATLAB Function2/2(referenceline_y_init) -> MATLAB Function4/2(referenceline_y_init)
  MATLAB Function2/1(referenceline_x_init) -> MATLAB Function4/1(referenceline_x_init)
  [host_x] -> mine_tou2/1(x_set)
  [host_y] -> mine_tou2/2(y_set)
  [global_path_y] -> mine_tou2/4(frenet_path_y_set)
  [global_path_x] -> mine_tou2/3(frenet_path_x_set)
  [global_path_x] -> MATLAB Function2/2(global_path_x)
  Bus Selector/7 -> [host_speed]  "<host_speed>"
  Bus Selector/6 -> [host_yawrate]  "<host_yawrate>"
  Bus Selector/5 -> [host_vy]  "<host_vy>"
  Bus Selector/4 -> [host_vx]  "<host_vx>"
  location info/1 -> Bus Selector/1
  Bus Selector/2 -> [host_y]  "<host_y>"
  Bus Selector/3 -> [host_heading_xy]  "<host_heading_xy>"
  Bus Selector/1 -> [host_x]  "<host_x>"
  Bus Selector1/1 -> [global_path_x]  "<global_path_x>"
  routine result/1 -> Bus Selector1/1
  Bus Selector1/2 -> [global_path_y]  "<global_path_y>"
  MATLAB Function4/1(referenceline_x) -> [referenceline_x]
  Bus Creator/1 -> Bus Creator1/1, referenceline info/1  "referenceline_info"
  [referenceline_x] -> Bus Creator/1  "referenceline_x"
  MATLAB Function4/2(referenceline_y) -> [referenceline_y]
  [referenceline_y] -> Bus Creator/2  "referenceline_y"
  Constant/1 -> [w_cost_smooth]
  Constant5/1 -> [y_lb]
  Constant4/1 -> [x_ub]
  Constant3/1 -> [x_lb]
  Constant2/1 -> [w_cost_ref]
  Constant1/1 -> [w_cost_length]
  Constant6/1 -> [y_ub]
  [w_cost_smooth] -> MATLAB Function4/3(w_cost_smooth)
  [w_cost_length] -> MATLAB Function4/4(w_cost_length)
  [w_cost_ref] -> MATLAB Function4/5(w_cost_ref)
  [x_lb] -> MATLAB Function4/6(x_lb)
  [x_ub] -> MATLAB Function4/7(x_ub)
  [y_lb] -> MATLAB Function4/8(y_lb)
  [y_ub] -> MATLAB Function4/9(y_ub)
  [host_match_point_index] -> Bus Creator1/2  "host_match_point_index"
  [w_cost_smooth] -> Bus Creator1/3  "w_cost_smooth"
  [w_cost_length] -> Bus Creator1/4  "w_cost_length"
  [w_cost_ref] -> Bus Creator1/5  "w_cost_ref"
  [x_lb] -> Bus Creator1/6  "x_lb"
  [x_ub] -> Bus Creator1/7  "x_ub"
  [y_lb] -> Bus Creator1/8  "y_lb"
  [y_ub] -> Bus Creator1/9  "y_ub"
  [reference_x_init] -> Bus Creator1/10  "reference_x_init"
  [reference_y_init] -> Bus Creator1/11  "reference_y_init"
  Bus Creator1/1 -> debug referenceline/1
  [referenceline_y] -> MATLAB Function3/2(path_y)
  [referenceline_x] -> MATLAB Function3/1(path_x)
  MATLAB Function3/1(path_heading) -> [referenceline_heading]
  MATLAB Function3/2(path_kappa) -> [referenceline_kappa]
  [referenceline_heading] -> Bus Creator/3  "reference_heading"
  [referenceline_kappa] -> Bus Creator/4  "reference_kappa"
  [host_x] -> mine_tou/1(x_set)
  [host_y] -> mine_tou/2(y_set)
  [referenceline_x] -> mine_tou/3(frenet_path_x_set)
  [referenceline_y] -> mine_tou/4(frenet_path_y_set)
  [referenceline_kappa] -> mine_tou/6(frenet_path_kappa_set)
  [referenceline_heading] -> mine_tou/5(frenet_path_heading_set)
  mine_tou/1(match_point_index_set) -> Selector1/1
  mine_tou/2(proj_x_set) -> Selector2/1
  mine_tou/3(proj_y_set) -> Selector3/1
  mine_tou/4(proj_heading_set) -> Selector4/1
  mine_tou/5(proj_kappa_set) -> Selector5/1
  Selector1/1 -> [origin_match_point_index]
  Selector2/1 -> [origin_x]
  Selector3/1 -> [origin_y]
  [origin_match_point_index] -> Bus Creator/5  "origin_match_point_index"
  [origin_x] -> Bus Creator/6  "origin_x"
  [origin_y] -> Bus Creator/7  "origin_y"
  mine_tou2/1(match_point_index_set) -> Selector/1
  Selector4/1 -> Terminator_1/1
  Selector5/1 -> Terminator_2/1
  mine_tou2/2(proj_x_set) -> Terminator_3/1
  mine_tou2/3(proj_y_set) -> Terminator_4/1
  mine_tou2/4(proj_heading_set) -> Terminator_5/1
  mine_tou2/5(proj_kappa_set) -> Terminator_6/1

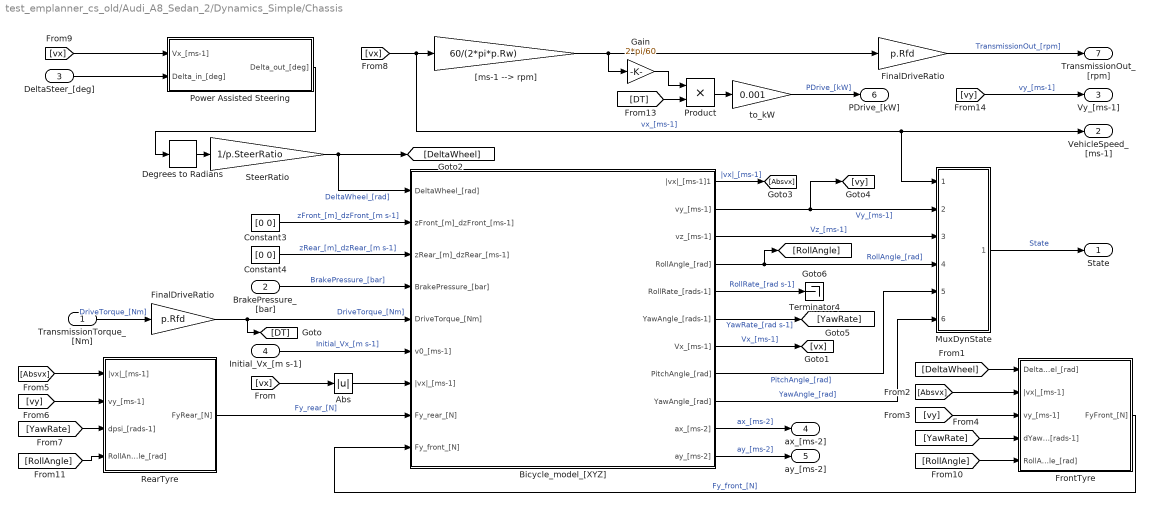
== system test_emplanner_cs_old/Audi_A8_Sedan_2/Dynamics_Simple/Chassis ==
  TransmissionTorque_[Nm] : Inport
  BrakePressure_[bar] : Inport  Port=2
  DeltaSteer_[deg] : Inport  Port=3
  Initial_Vx_[m s-1] : Inport  Port=4
  Abs : Abs
  Bicycle_model_[XYZ] : Subsystem
      mask Display: image(imread('Bicycle_model.png'));
  Constant3 : Constant  Value=[0 0]
  Constant4 : Constant  Value=[0 0]
  Degrees to Radians : simulink_extras/Transformations/Degrees to Radians
  FinalDriveRatio : Gain  Gain=p.Rfd  SaturateOnIntegerOverflow=on  OutDataTypeStr=Inherit: Same as input  ParamDataTypeStr=Inherit: Same as input
  "FinalDriveRatio " : Gain  Gain=p.Rfd  SaturateOnIntegerOverflow=on  OutDataTypeStr=Inherit: Same as input  ParamDataTypeStr=Inherit: Same as input
  FrontTyre : Subsystem
      mask Display: image(imread('Tyre.png'));
  Gain : Gain  Gain=2*pi/60
  MuxDynState : Subsystem
  Power Assisted Steering : Subsystem
  Product : Product  RndMeth=Zero
  RearTyre : Subsystem
      mask Display: image(imread('Tyre.png'));
  SteerRatio : Gain  Gain=1/p.SteerRatio
  Terminator4 : Terminator
  "[ms-1 --> rpm]" : Gain  Gain=60/(2*pi*p.Rw)  SaturateOnIntegerOverflow=on  OutDataTypeStr=Inherit: Same as input  ParamDataTypeStr=Inherit: Same as input
  to_kW : Gain  Gain=0.001
  State : Outport
  VehicleSpeed_[ms-1] : Outport  Port=2
  Vy_[ms-1] : Outport  Port=3
  ax_[ms-2] : Outport  Port=4
  ay_[ms-2] : Outport  Port=5
  PDrive_[kW] : Outport  Port=6
  TransmissionOut_[rpm] : Outport  Port=7
  wires:
  [vy] -> Vy_[ms-1]/1  "vy_[ms-1]"
  to_kW/1 -> PDrive_[kW]/1  "PDrive_[kW]"
  Gain/1 -> Product/1
  Bicycle_model_[XYZ]/10(ax_[ms-2]) -> ax_[ms-2]/1  "ax_[ms-2]"
  Product/1 -> to_kW/1
  [DT] -> Product/2
  Bicycle_model_[XYZ]/11(ay_[ms-2]) -> ay_[ms-2]/1  "ay_[ms-2]"
  Abs/1 -> Bicycle_model_[XYZ]/7(|vx|_[ms-1])
  Degrees to Radians/1 -> SteerRatio/1
  [vx] -> Abs/1
  SteerRatio/1 -> [DeltaWheel], Bicycle_model_[XYZ]/1(DeltaWheel_[rad])  "DeltaWheel_[rad]"
  TransmissionTorque_[Nm]/1 -> "FinalDriveRatio "/1  "DriveTorque_[Nm]"
  RearTyre/1(FyRear_[N]) -> Bicycle_model_[XYZ]/8(Fy_rear_[N])  "Fy_rear_[N]"
  FrontTyre/1(FyFront_[N]) -> Bicycle_model_[XYZ]/9(Fy_front_[N])  "Fy_front_[N]"
  Bicycle_model_[XYZ]/1(|vx|_[ms-1]1) -> [Absvx]  "|vx|_[ms-1]"
  Bicycle_model_[XYZ]/2(vy_[ms-1]) -> [vy], MuxDynState/2(vy [ms-1])  "Vy_[ms-1]"
  Bicycle_model_[XYZ]/4(RollAngle_[rad]) -> MuxDynState/4(R [rad]), [RollAngle]  "RollAngle_[rad]"
  Bicycle_model_[XYZ]/6(YawAngle_[rads-1]) -> [YawRate]  "YawRate_[rad s-1]"
  Bicycle_model_[XYZ]/7(Vx_[ms-1]) -> [vx]  "Vx_[ms-1]"
  [DeltaWheel] -> FrontTyre/1(DeltaWheel_[rad])
  [Absvx] -> FrontTyre/2(|vx|_[ms-1])
  [vy] -> FrontTyre/3(vy_[ms-1])
  [YawRate] -> FrontTyre/4(dYawAngle_[rads-1])
  [Absvx] -> RearTyre/1(|vx|_[ms-1])
  [vy] -> RearTyre/2(vy_[ms-1])
  [YawRate] -> RearTyre/3(dpsi_[rads-1])
  Bicycle_model_[XYZ]/3(vz_[ms-1]) -> MuxDynState/3(vz [ms-1])  "Vz_[ms-1]"
  Bicycle_model_[XYZ]/8(PitchAngle_[rad]) -> MuxDynState/5(P [rad])  "PitchAngle_[rad]"
  Bicycle_model_[XYZ]/9(YawAngle_[rad]) -> MuxDynState/6(Y [rad])  "YawAngle_[rad]"
  "[ms-1 --> rpm]"/1 -> Gain/1, FinalDriveRatio/1
  FinalDriveRatio/1 -> TransmissionOut_[rpm]/1  "TransmissionOut_[rpm]"
  [vx] -> "[ms-1 --> rpm]"/1, VehicleSpeed_[ms-1]/1, MuxDynState/1(vx [ms-1])  "vx_[ms-1]"
  [vx] -> Power Assisted Steering/1(Vx_[ms-1])
  DeltaSteer_[deg]/1 -> Power Assisted Steering/2(Delta_in_[deg])
  Power Assisted Steering/1(Delta_out_[deg]) -> Degrees to Radians/1
  [RollAngle] -> FrontTyre/5(RollAngle_[rad])
  [RollAngle] -> RearTyre/4(RollAngle_[rad])
  Constant3/1 -> Bicycle_model_[XYZ]/2(zFront_[m]_dzFront_[ms-1])  "zFront_[m]_dzFront_[m s-1]"
  Constant4/1 -> Bicycle_model_[XYZ]/3(zRear_[m]_dzRear_[ms-1])  "zRear_[m]_dzRear_[m s-1]"
  BrakePressure_[bar]/1 -> Bicycle_model_[XYZ]/4(BrakePressure_[bar])  "BrakePressure_[bar]"
  "FinalDriveRatio "/1 -> Bicycle_model_[XYZ]/5(DriveTorque_[Nm]), [DT]  "DriveTorque_[Nm]"
  Initial_Vx_[m s-1]/1 -> Bicycle_model_[XYZ]/6(v0_[ms-1])  "Initial_Vx_[m s-1]"
  Bicycle_model_[XYZ]/5(RollRate_[rads-1]) -> Terminator4/1  "RollRate_[rad s-1]"
  MuxDynState/1(State) -> State/1  "State"

== system test_emplanner_cs_old/Audi_A8_Sedan_2/Dynamics_Simple/Engine ==
  ImpellerTorque_[Nm] : Inport
  Throttle_[%] : Inport  Port=2
  Configurable Subsystem : Subsystem  BlockChoice=Rate Limiter  mask{ComputationMode=ComputationMode}
      mask prompts: ComputationMode "Compuation mode:"
      mask init:
      | SetComputationMode(gcb,ComputationMode);
      settings: AttributesFormatString=%<BlockChoice>  OpenFcn=BringToFront(gcb);  MemberBlocks=Discrete Rate Limiter,Rate Limiter
      settings: TemplateBlock=|
      | PreScanSimulinkLibrary/Configurable Subsystems/TransferFunction
      | Engine/Configurable
      | Subsystem
  Configurable Subsystem1 : Subsystem  BlockChoice=Integrator  mask{ComputationMode=ComputationMode}
      mask prompts: ComputationMode "Computation mode:"
      mask init:
      | SetComputationMode(gcb,ComputationMode);
      settings: AttributesFormatString=%<BlockChoice>  OpenFcn=BringToFront(gcb);  MemberBlocks=Discrete-Time Integrator,Integrator
      settings: TemplateBlock=|
      | PreScanSimulinkLibrary/Configurable Subsystems/integral with initial condition and limts
      | for engine/Configurable
      | Subsystem
  EngineTorque : Lookup2D  RowIndex=p.thvec  ColumnIndex=p.nevec  Table=p.emap  InputSameDT=on
  Gain : Gain  Gain=2*pi/60
  Product : Product  RndMeth=Zero
  Sum : Sum  Inputs=-+  InputSameDT=on  SaturateOnIntegerOverflow=on  OutDataTypeStr=Inherit: Same as first input
  engine + impeller inertia : Gain  Gain=1/p.Iei  SaturateOnIntegerOverflow=on  OutDataTypeStr=Inherit: Same as input  ParamDataTypeStr=Inherit: Same as input
  rad|sec2rpm : Gain  Gain=60/2/pi  SaturateOnIntegerOverflow=on  OutDataTypeStr=Inherit: Same as input  ParamDataTypeStr=Inherit: Same as input
  to_kW : Gain  Gain=0.001
  nEngine_[rpm] : Outport  InitialOutput=0
  PEngine_[kW] : Outport  Port=2  InitialOutput=0
  wires:
  rad|sec2rpm/1 -> nEngine_[rpm]/1, EngineTorque/2, Gain/1  "rpm"
  engine + impeller inertia/1 -> Configurable Subsystem1/1(In1)  "rads-2"
  EngineTorque/1 -> Sum/2, Product/2
  Sum/1 -> engine + impeller inertia/1
  Configurable Subsystem1/1(Out1) -> rad|sec2rpm/1  "rads-1"
  Throttle_[%]/1 -> Configurable Subsystem/1(In1)
  ImpellerTorque_[Nm]/1 -> Sum/1
  Configurable Subsystem/1(Out1) -> EngineTorque/1
  Product/1 -> to_kW/1
  Gain/1 -> Product/1
  to_kW/1 -> PEngine_[kW]/1

== system test_emplanner_cs_old/Audi_A8_Sedan_2/Dynamics_Simple/Gear: Auto Manual ==
  note: 0; Auto = on // Manual =off
      | 1; Auto = off // Manual =on
  Auto_Manual : Inport
  Manual_Gear : Inport  Port=2
  Auto_Gear : Inport  Port=3
  If : If  IfExpression=u1 == 0
  If Action Subsystem : Subsystem  TreatAsAtomicUnit=on
  If Action Subsystem1 : Subsystem  TreatAsAtomicUnit=on
  Merge : Merge
  Gear : Outport
  wires:
  If Action Subsystem/1(Out1) -> Merge/1
  Auto_Gear/1 -> If Action Subsystem/1(In1)
  If/1 -> If Action Subsystem/Action
  Merge/1 -> Gear/1
  If Action Subsystem1/1(Out1) -> Merge/2
  Manual_Gear/1 -> If Action Subsystem1/1(In1)
  If/2 -> If Action Subsystem1/Action
  Auto_Manual/1 -> If/1

== system test_emplanner_cs_old/Audi_A8_Sedan_2/Dynamics_Simple/ShiftLogic ==
  Throttle_[%] : Inport
  GearNr_[-] : Inport  Port=2
  Auto_GearShift : Inport  Port=3
  VehSpeed_[ms-1] : Inport  Port=4
  Add2 : Sum
  Data Type Conversion1 : DataTypeConversion  OutDataTypeStr=double
  Detect Increase1 : simulink/Logic and Bit Operations/Detect Increase  vinit=0.0  OutDataTypeStr=uint8
  Detect Increase : Subsystem
  Gear limitation : Saturate  UpperLimit=p.maxGear  LowerLimit=1
  Gear limitation while shifting : Saturate  UpperLimit=p.maxGear  LowerLimit=1
  GearNeutral : Constant  Value=0
  GearReverse : Constant  Value=-1
  "IC, gear = 1" : Memory  InitialCondition=1  InheritSampleTime=on
  If Action Neutral : Subsystem  TreatAsAtomicUnit=on
  If Action Normal : Subsystem  TreatAsAtomicUnit=on
  If Action Reverse : Subsystem  TreatAsAtomicUnit=on
  Memory : Memory  InheritSampleTime=on
  Merge : Merge  Inputs=3
  Relational Operator : RelationalOperator  OutDataTypeStr=boolean  RndMeth=Nearest
  Relational Operator1 : RelationalOperator  Operator=<=  OutDataTypeStr=boolean  RndMeth=Nearest
  Shift_Down time : Delay  DelayLength=p.ShiftDown_fac
  Shift_Up time : Delay  DelayLength=p.ShiftUp_fac
  Sum : Sum  Inputs=+-
  interp_down : Lookup2D  RowIndex=p.downth  ColumnIndex=[1:p.maxGear]  Table=p.downtab  LookUpMeth=Interpolation-Use End Values  InputSameDT=on
  interp_up : Lookup2D  RowIndex=p.upth  ColumnIndex=[1:p.maxGear]  Table=p.uptab  LookUpMeth=Interpolation-Use End Values  InputSameDT=on
  reverse/neutral/normal gear : If  IfExpression=u1 == 0  ElseIfExpressions=u1 < 0
  to_ms-1 : Gain  Gain=1/3.6
  "to_ms-1 " : Gain  Gain=1/3.6
  GearNr : Outport
  wires:
  Auto_GearShift/1 -> reverse/neutral/normal gear/1
  "IC, gear = 1"/1 -> If Action Normal/1(In1)
  Merge/1 -> GearNr/1
  If Action Reverse/1(Out1) -> Merge/2
  If Action Neutral/1(Out1) -> Merge/1
  If Action Normal/1(Out1) -> Merge/3
  reverse/neutral/normal gear/3 -> If Action Normal/Action
  reverse/neutral/normal gear/1 -> If Action Neutral/Action
  reverse/neutral/normal gear/2 -> If Action Reverse/Action
  GearReverse/1 -> If Action Reverse/1(In1)
  GearNeutral/1 -> If Action Neutral/1(In1)
  Shift_Down time/1 -> Sum/2
  Shift_Up time/1 -> Sum/1
  Detect Increase/1(Out1) -> Shift_Up time/1
  Data Type Conversion1/1 -> Shift_Down time/1
  Detect Increase1/1 -> Data Type Conversion1/1
  Sum/1 -> Add2/1
  Memory/1 -> Add2/2  "GearNr_[-]"
  Add2/1 -> Gear limitation while shifting/1
  Gear limitation while shifting/1 -> "IC, gear = 1"/1, Memory/1  "GearNr_[-]"
  Throttle_[%]/1 -> interp_down/1, interp_up/1
  Relational Operator/1 -> Detect Increase/2(In2)
  Relational Operator1/1 -> Detect Increase1/1
  interp_down/1 -> "to_ms-1 "/1
  VehSpeed_[ms-1]/1 -> Relational Operator/1, Relational Operator1/1
  interp_up/1 -> to_ms-1/1
  Gear limitation/1 -> interp_down/2, interp_up/2, Detect Increase/1(GearNr_[-])
  GearNr_[-]/1 -> Gear limitation/1
  to_ms-1/1 -> Relational Operator/2
  "to_ms-1 "/1 -> Relational Operator1/2

== system test_emplanner_cs_old/Audi_A8_Sedan_2/Dynamics_Simple/Transmission ==
  nEngine_[rpm] : Inport
  GearNr_[-] : Inport  Port=2
  n_TransmissionOut_[rpm] : Inport  Port=3
  Torque_Converter : Subsystem
      mask Display: image(imread('TorqueConverter.png'));
  Transmission_Ratio : Subsystem
  Viscous coupling : Lookup  InputValues=[-5:0.1:5]*p.m/4  Table=p.m/4*tanh([-5:0.1:5])
  ImpellerTorque_[Nm] : Outport  InitialOutput=0
  TransmissionTorque_[Nm] : Outport  Port=2  InitialOutput=0
  wires:
  Torque_Converter/2(TurbineTorque_[Nm]) -> Viscous coupling/1  "Converter_Torque_[Nm]"
  Transmission_Ratio/2(nTransmissionIn_[rpm]) -> Torque_Converter/2(nTransmission_[rpm])
  nEngine_[rpm]/1 -> Torque_Converter/1(nEngine_[rpm])
  GearNr_[-]/1 -> Transmission_Ratio/2(GearNr_[-]), Torque_Converter/3(Gear nr)
  n_TransmissionOut_[rpm]/1 -> Transmission_Ratio/3(nTransmissionOut_[rpm])
  Torque_Converter/1(ImpellerTorque_[Nm]) -> ImpellerTorque_[Nm]/1
  Transmission_Ratio/1(tTransmissionOut_[Nm]) -> TransmissionTorque_[Nm]/1
  Viscous coupling/1 -> Transmission_Ratio/1(tTransmissionIn_[Nm])

== system test_emplanner_cs_old/Audi_A8_Sedan_2/PathFollower_Preview_1/LateralController ==
  TrajOffset x,y,Y [m,m,deg] : Inport
  ActorOffset_Left(+) / Right(-) [m] : Inport  Port=2
  position x,y,Y [m,m,deg] : Inport  Port=3
  vx [m/s] : Inport  Port=4
  vy [m/s] : Inport  Port=5
  Yaw rate [deg/s] : Inport  Port=6
  CorneringStiffness_Tyres_Front [N/rad] : Inport  Port=7
  CorneringStiffness_Tyres_Rear [N/rad] : Inport  Port=8
  steering_ratio[-] : Inport  Port=9
  Avoid_0 : Saturate  UpperLimit=1000  LowerLimit=0.1
  CTRL REFERENCES : Subsystem
  Calculate delta steering error : Subsystem
      mask Display:
      | port_label('input', 1, 'v_x_vehicle [m/s]')
      | port_label('input', 2, 'v_x_vehicle_Min [m/s]')
      | port_label('input', 3, 't_Preview_LatCtrl [s]')
      | port_label('input', 4, 'v_y_vehicle [m/s]')
      | port_label('input', 5, 'yawrate_vehicle [rad/sec]')
      | port_label('input', 6, 'CorneringStiffness_Tyres_Front [N/rad]')
      | port_label('input', 7, 'CorneringStiffness_Tyres_Rear [N/rad]')
      | port_label('input', 8, 'm_vehicle_total [kg]')
      | port_label('input', 9, 'inertia_z_vehicle_total [kg m2]')
      | port_label('input', 10, 'e_Lat [m]')
      | port_label('input', 11, 'Distance_frontaxle_COG(+) [m]')
      | port_label('input', 12, 'wheel_base [m]')
      | port_label('output', 1, 'delta_steeringwheel [rad]')
  Const_t_Preview_LatCtrl[s] : Constant  Value=PreviewTime  SampleTime=CSSampleTime
  Const_v_x_Vehicle_Min[km|h] : Constant  Value=LowSpeedLimit  SampleTime=CSSampleTime
  Constant6 : Constant  SampleTime=CSSampleTime
  Demux : Demux  Outputs=3
  Demux1 : Demux  Outputs=3
  Distance_frontaxle_COG(+) [m] : Constant  Value=length_a  SampleTime=CSSampleTime
  Gain : Gain  Gain=1*pi/180
  Gain1 : Gain  Gain=1*pi/180
  Gain4 : Gain
  Memory : Memory  InheritSampleTime=on
  Memory1 : Memory  InheritSampleTime=on
  Memory2 : Memory  InheritSampleTime=on
  Mux : Mux  Inputs=3
  Mux1 : Mux  Inputs=3
  SteeringWheelAngle : Subsystem
  deg to rad : Gain  Gain=pi/180
  inertia_z_vehicle_total [kg m2] : Constant  Value=Jzz  SampleTime=CSSampleTime
  km|h to m|s : Gain  Gain=1/3.6
  m_vehicle_total_[kg] : Constant  Value=mass  SampleTime=CSSampleTime
  s_Preview_LatCtrl : Subsystem
  wheel_base [m] : Constant  Value=length_l  SampleTime=CSSampleTime
  Actor/Traj_distance [m] : Outport
  Actor/Traj_angle [deg] : Outport  Port=2
  delta_steerwheel [deg] : Outport  Port=3
  wires:
  km|h to m|s/1 -> Calculate delta steering error/2(In2), s_Preview_LatCtrl/2(v_x_Vehicle_Min[m|s])
  Gain/1 -> Mux/3
  Mux/1 -> CTRL REFERENCES/3(TrajOffset [m,m,rad])
  ActorOffset_Left(+) / Right(-) [m]/1 -> CTRL REFERENCES/4(ActorOffset_Left(+) / Right(-)_[m])
  Demux/1 -> Mux/1
  Demux/2 -> Mux/2
  Demux/3 -> Gain/1
  TrajOffset x,y,Y [m,m,deg]/1 -> Demux/1
  CTRL REFERENCES/2(Actor/Traj_angle [deg]) -> Actor/Traj_angle [deg]/1
  CTRL REFERENCES/1(Actor/Traj_distance [m]) -> Actor/Traj_distance [m]/1
  Calculate delta steering error/1(Out1) -> SteeringWheelAngle/1(Angle_Steering[rad])
  vx [m/s]/1 -> Memory1/1
  vy [m/s]/1 -> Memory2/1
  CorneringStiffness_Tyres_Front [N/rad]/1 -> Calculate delta steering error/6(In6)
  m_vehicle_total_[kg]/1 -> Calculate delta steering error/8(In8)
  inertia_z_vehicle_total [kg m2]/1 -> Calculate delta steering error/9(In9)
  steering_ratio[-]/1 -> SteeringWheelAngle/2(i_Steering[])
  SteeringWheelAngle/1(Angle_SteeringWheel[deg]) -> Gain4/1, Memory/1
  Memory/1 -> SteeringWheelAngle/3(Angle_SteeringWheel_Last[deg])
  Constant6/1 -> SteeringWheelAngle/4(LatCtrl1_Enable[0Off|1On])
  Avoid_0/1 -> Calculate delta steering error/3(In3), s_Preview_LatCtrl/3(t_Preview_LatCtrl[s])
  Const_v_x_Vehicle_Min[km|h]/1 -> km|h to m|s/1
  s_Preview_LatCtrl/1(s_Preview_LatCtrl[m]) -> CTRL REFERENCES/2(Position Preview Distance [m])
  Const_t_Preview_LatCtrl[s]/1 -> Avoid_0/1
  Gain4/1 -> delta_steerwheel [deg]/1
  Distance_frontaxle_COG(+) [m]/1 -> Calculate delta steering error/11(In11)
  CorneringStiffness_Tyres_Rear [N/rad]/1 -> Calculate delta steering error/7(In7)
  Yaw rate [deg/s]/1 -> deg to rad/1
  deg to rad/1 -> Calculate delta steering error/5(In5)
  Gain1/1 -> Mux1/3
  Demux1/1 -> Mux1/1
  Demux1/2 -> Mux1/2
  Demux1/3 -> Gain1/1
  position x,y,Y [m,m,deg]/1 -> Demux1/1
  Mux1/1 -> CTRL REFERENCES/1(Pos x,y,Y [m,m,rad])
  wheel_base [m]/1 -> Calculate delta steering error/12(In12)
  CTRL REFERENCES/3(e_Lat [m]) -> Calculate delta steering error/10(In10)
  Memory1/1 -> Calculate delta steering error/1(In1), s_Preview_LatCtrl/1(v_x_Vehicle[m|s])
  Memory2/1 -> Calculate delta steering error/4(In4)
